simulink model "Sample"  (R2020a)
settings: Solver=FixedStepAuto  StartTime=0.0  StopTime=Inf  RelTol=1e-3  EnableMultiTasking=on
settings Model: Creator=eisuk  LastModifiedBy=eisuk
settings SolverCC: PositivePriorityOrder=on
settings DataIOCC: ReturnWorkspaceOutputs=off
settings OptimizationCC: EnhancedBackFolding=on  PassReuseOutputArgsAs=Individual arguments  ZeroExternalMemoryAtStartup=off  ZeroInternalMemoryAtStartup=off  MaxStackSize=64  OptimizeBlockOrder=speed  DifferentSizesBufferReuse=on  OptimizationCustomize=off  EfficientTunableParamExpr=on
settings DebuggingCC: ParameterTunabilityLossMsg=error
settings HardwareCC: ProdBitPerPointer=32  ProdBitPerSizeT=32  ProdBitPerPtrDiffT=32  ProdLargestAtomicInteger=Long  ProdLargestAtomicFloat=Double  ProdWordSize=32  ProdLongLongMode=on  ProdHWDeviceType=ARM Compatible->ARM Cortex
settings RTWCC: SystemTargetFile=ert.tlc  HardwareBoard=Raspberry Pi  TemplateMakefile=ert_default_tmf  Toolchain=GNU GCC Raspberry Pi  BuildConfiguration=Faster Runs
settings CodeAppCC: ForceParamTrailComments=on  IgnoreCustomStorageClasses=off  OperatorAnnotations=on  SimulinkDataObjDesc=on  SFDataObjDesc=on  InsertBlockDesc=on
settings ERTTargetCC: SupportVariableSizeSignals=on

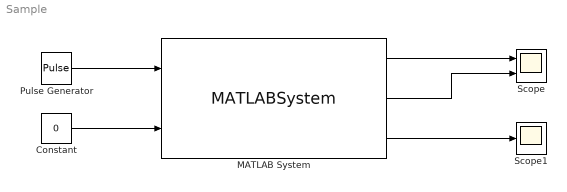
== system Sample ==
  Constant : Constant  Value=0
  MATLAB System : MATLABSystem  System=RoboClawDriver  tty=/dev/ttyACM0  baudrate=38400  mode=Speed  SampleTime=0.01  address=128 (0x80)  timeout=0  retries=30  strict_0xFF_ACK=0
      mask Type: RoboClawDriver
      mask Display:
      | disp(['RoboClaw' char(10) '' char(10) 'Port : /dev/ttyACM0' char(10) 'Baudrate : 38400bps']);
      | port_label('input',1,'M1 Speed');
      | port_label('input',2,'M2 Speed');
      | port_label('output',1,'M1 Encoder');
      | port_label('output',2,'M2 Encoder');
      | port_label('output',3,'Main battery');
  Pulse Generator : DiscretePulseGenerator  Period=200  PulseWidth=50  PhaseDelay=100  SampleTime=0.01
  Scope : Scope  NumInputPorts=2
  Scope1 : Scope
  wires:
  MATLAB System/1 -> Scope/1
  MATLAB System/2 -> Scope/2
  MATLAB System/3 -> Scope1/1
  Constant/1 -> MATLAB System/2
  Pulse Generator/1 -> MATLAB System/1
